simulink library "INT_CoEng_StEng"  (R2016b)
settings: Solver=VariableStepAuto  StartTime=0.0  StopTime=10.0  RelTol=1e-3
settings Model: Creator=zhoutinglin  LastModifiedBy=zhoutinglin

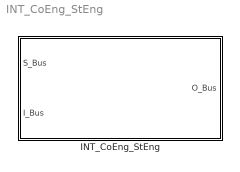
== system INT_CoEng_StEng ==
  INT_CoEng_StEng : Subsystem

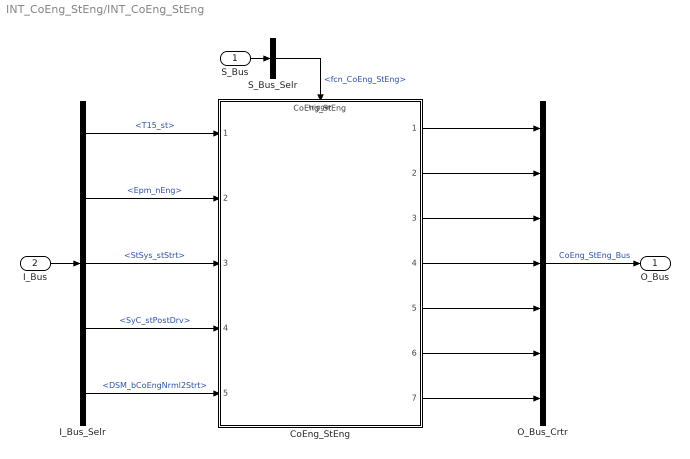
== system INT_CoEng_StEng/INT_CoEng_StEng ==
  S_Bus : Inport
  I_Bus : Inport  Port=2
  CoEng_StEng : ModelReference  ModelNameDialog=CoEng_StEng  SimulationMode=Normal  ModelReferenceVersion=1.61  TriggerPortName=function  TriggerPortTriggerType=function-call  TriggerPortStatesWhenEnabling=held
  I_Bus_Selr : BusSelector  OutputSignals=T15_st,Epm_nEng,StSys_stStrt,SyC_stPostDrv,DSM_bCoEngNrml2Strt
  O_Bus_Crtr : BusCreator  Inputs=7
  S_Bus_Selr : BusSelector  OutputSignals=fcn_CoEng_StEng
  O_Bus : Outport
  wires:
  S_Bus_Selr/1 -> CoEng_StEng/Trigger  "<fcn_CoEng_StEng>"
  S_Bus/1 -> S_Bus_Selr/1
  I_Bus/1 -> I_Bus_Selr/1
  I_Bus_Selr/1 -> CoEng_StEng/1  "<T15_st>"
  I_Bus_Selr/2 -> CoEng_StEng/2  "<Epm_nEng>"
  I_Bus_Selr/3 -> CoEng_StEng/3  "<StSys_stStrt>"
  I_Bus_Selr/4 -> CoEng_StEng/4  "<SyC_stPostDrv>"
  I_Bus_Selr/5 -> CoEng_StEng/5  "<DSM_bCoEngNrml2Strt>"
  O_Bus_Crtr/1 -> O_Bus/1  "CoEng_StEng_Bus"
  CoEng_StEng/1 -> O_Bus_Crtr/1
  CoEng_StEng/2 -> O_Bus_Crtr/2
  CoEng_StEng/3 -> O_Bus_Crtr/3
  CoEng_StEng/4 -> O_Bus_Crtr/4
  CoEng_StEng/5 -> O_Bus_Crtr/5
  CoEng_StEng/6 -> O_Bus_Crtr/6
  CoEng_StEng/7 -> O_Bus_Crtr/7
